simulink model "Counter_Down"  (R2018a)
settings: Solver=VariableStepAuto  StartTime=0.0  StopTime=10.0  RelTol=1e-3
settings Model: Creator=user  LastModifiedBy=user

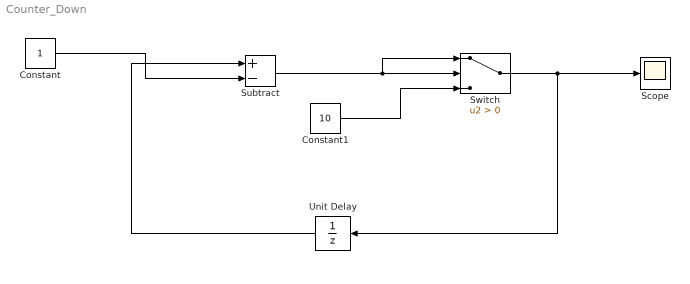
== system Counter_Down ==
  Constant : Constant
  Constant1 : Constant  Value=10
  Scope : Scope
  Subtract : Sum  Inputs=+-
  Switch : Switch  Criteria=u2 > Threshold
  Unit Delay : UnitDelay  SampleTime=-1
  wires:
  Constant/1 -> Subtract/2
  Constant1/1 -> Switch/3
  Subtract/1 -> Switch/1, Switch/2
  Unit Delay/1 -> Subtract/1
  Switch/1 -> Unit Delay/1, Scope/1
